simulink library "Lib_Turbo_ValvePHY_TMATS_new"  (R2015a)
settings: Solver=ode45  StartTime=0.0  StopTime=10.0  RelTol=1e-3
Description:
  | Thomas Modules
settings Model: Creator=jwchapm2  LastModifiedBy=jwhitfie
settings OptimizationCC: ExpressionDepthLimit=2147483647
settings DebuggingCC: UnderspecifiedInitializationDetection=Classic  MergeDetectMultiDrivingBlocksExec=none  SolverPrmCheckMsg=warning  StateNameClashWarn=warning

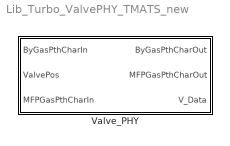
== system Lib_Turbo_ValvePHY_TMATS_new ==
  Valve_PHY : Subsystem  mask(T-MATS: Valve_Phy Library Block){s_V_AeVLV_M=200, s_V_AeBYP_M=200, s_V_AeTH_M=167, X_V_FARVec_M=[0 1], T_V_RtVec_M=[0 .99], Y_V_TtVec_M=[1 10000], T_V_gammaArray_M=[1.4 1.4; 1.4 1.4]}
      mask prompts: s_V_AeVLV_M "s_V_AeVLV_M - Valve area [in^2]"; s_V_AeBYP_M "s_V_AeBYP_M - Valve bypass area [in^2]"; s_V_AeTH_M "s_V_AeTH_M - Valve throat area [in^2]"; X_V_FARVec_M "X_V_FARVec_M - Fuel to Air ratio (x - axis) [frac]"; T_V_RtVec_M "T_V_RtVec_M - R Array (Rt = f(FAR))"; Y_V_TtVec_M "Y_V_TtVec_M - Total Temperature Vector (y - axis) [degR]"; T_V_gammaArray_M "T_V_gammaArray_M - Gamma Array (Gamma = f(FAR, Tt))"
      mask help: This block simulates the performance of a valve using basic thermodynamic equations, properties, and table lookups.
      mask Help: web(which('Turbo_TMATS_VlvPHY.html'),'-helpbrowser')

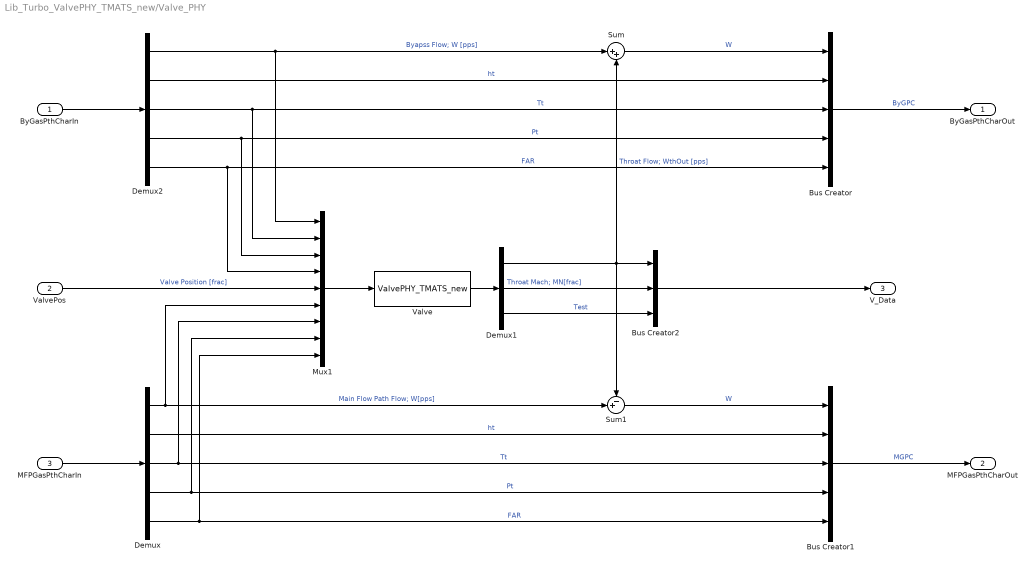
== system Lib_Turbo_ValvePHY_TMATS_new/Valve_PHY ==
  ByGasPthCharIn : Inport
  ValvePos : Inport  Port=2
  MFPGasPthCharIn : Inport  Port=3
  Bus Creator : BusCreator  Inputs=5
  Bus Creator1 : BusCreator  Inputs=5
  Bus Creator2 : BusCreator  Inputs=3
  Demux : Demux  Outputs=5
  Demux1 : Demux  Outputs=3
  Demux2 : Demux  Outputs=5
  Mux1 : Mux  Inputs=9
  Sum : Sum  Inputs=|++
  Sum1 : Sum  Inputs=-+|
  Valve : S-Function  FunctionName=ValvePHY_TMATS_new  Parameters=s_V_AeVLV_M, s_V_AeBYP_M, s_V_AeTH_M, X_V_FARVec_M, T_V_RtVec_M, Y_V_TtVec_M, T_V_gammaArray_M, gcs  SFunctionModules='interp1Ac_TMATS interp2Ac_TMATS calc_Pstatic_TMATS calc_WvsMN_TMATS calc_PsvsMN_TMATS functions_TMATS'
  ByGasPthCharOut : Outport
  MFPGasPthCharOut : Outport  Port=2
  V_Data : Outport  Port=3
  wires:
  Bus Creator1/1 -> MFPGasPthCharOut/1  "MGPC"
  MFPGasPthCharIn/1 -> Demux/1
  Demux/5 -> Mux1/9, Bus Creator1/5  "FAR"
  Demux/3 -> Mux1/7, Bus Creator1/3  "Tt"
  Demux/4 -> Mux1/8, Bus Creator1/4  "Pt"
  Mux1/1 -> Valve/1
  Demux/1 -> Mux1/6, Sum1/2  "Main Flow Path Flow; W[pps]"
  Demux1/1 -> Sum/2, Bus Creator2/1, Sum1/1  "Throat Flow; WthOut [pps]"
  Valve/1 -> Demux1/1
  ByGasPthCharIn/1 -> Demux2/1
  Demux2/4 -> Mux1/3, Bus Creator/4  "Pt"
  Sum/1 -> Bus Creator/1  "W"
  Demux2/1 -> Mux1/1, Sum/1  "Byapss Flow; W [pps]"
  Sum1/1 -> Bus Creator1/1  "W"
  Demux2/5 -> Mux1/4, Bus Creator/5  "FAR"
  Demux2/3 -> Mux1/2, Bus Creator/3  "Tt"
  Bus Creator/1 -> ByGasPthCharOut/1  "ByGPC"
  Demux1/3 -> Bus Creator2/3  "Test"
  Bus Creator2/1 -> V_Data/1
  Demux2/2 -> Bus Creator/2  "ht"
  Demux/2 -> Bus Creator1/2  "ht"
  ValvePos/1 -> Mux1/5  "Valve Position [frac]"
  Demux1/2 -> Bus Creator2/2  "Throat Mach; MN[frac]"
